simulink model "ros2webots_localization_model"  (R2023a)
settings: Solver=FixedStepAuto  StartTime=0.0  StopTime=inf  FixedStep=0.05  RelTol=1e-3  EnableMultiTasking=on
model workspace (MAT data in the model file):
  Logfile_Data_Object = robotics.ros.BagSelection
  Logfile_Data_Object.FilePath = '\\wsl.localhost\ubuntu\home\mjavadzallaghi\ros2_ws\ros2webots\baglog\rosbot_data_20240125_225927.bag'
  Logfile_Data_Object.StartTime = 1706210981.23
  Logfile_Data_Object.EndTime = 1706211126.25
  Logfile_Data_Object.NumMessages = 508
  Logfile_Data_Object.AvailableTopics = table
  Logfile_Data_Object.AvailableTopics.data{1} = [73; 435]
  Logfile_Data_Object.AvailableTopics.data{2} = categorical
  Logfile_Data_Object.AvailableTopics.data{2}.categoryNames = {'geometry_msgs/Twist'; 'sensor_msgs/Imu'}
  Logfile_Data_Object.AvailableTopics.data{2}.codes = [1; 2]
  Logfile_Data_Object.AvailableTopics.data{3}{1} = 'geometry_msgs/Vector3 Linear
    |   double X
    |   double Y
    |   double Z
    | geometry_msgs/Vector3 Angular
    |   double X
    |   double Y
    |   double Z
    | '
  Logfile_Data_Object.AvailableTopics.data{3}{2} = 'std_msgs/Header Header
    |   uint32 Seq
    |   Time Stamp
    |   char FrameId
    | geometry_msgs/Quaternion Orientation
    |   double X
    |   double Y
    |   double Z
    |   double W
    | double[9] OrientationCovariance
    | geometry_msgs/Vector3 AngularVelocity
    |   double X
    |   double Y
    |   double Z
    | double[9] AngularVelocityCovariance
    | geometry_msgs/Vector3 LinearAcceleration
    |   double X
    |   double Y
    |   double Z
    | double[9] LinearAccelerationCovariance
    | '
  Logfile_Data_Object.AvailableTopics.ndims = 2
  Logfile_Data_Object.AvailableTopics.nrows = 2
  Logfile_Data_Object.AvailableTopics.rownames = {'/webots/rosbot/command_vel'; '/webots/rosbot/imu'}
  Logfile_Data_Object.AvailableTopics.nvars = 3
  Logfile_Data_Object.AvailableTopics.varnames = {'NumMessages', 'MessageType', 'MessageDefinition'}
  Logfile_Data_Object.AvailableTopics.props.useVariableNamesOriginal = 0
  Logfile_Data_Object.AvailableTopics.props.useDimensionNamesOriginal = 0
  Logfile_Data_Object.AvailableTopics.props.CustomProps = struct()
  Logfile_Data_Object.AvailableTopics.props.VariableCustomProps = struct()
  Logfile_Data_Object.AvailableTopics.props.versionSavedFrom = 4
  Logfile_Data_Object.AvailableTopics.props.minCompatibleVersion = 1
  Logfile_Data_Object.AvailableTopics.props.incompatibilityMsg = ''
  Logfile_Data_Object.AvailableTopics.props.VersionSavedFrom = 4
  Logfile_Data_Object.AvailableTopics.props.Description = ''
  Logfile_Data_Object.AvailableTopics.props.VariableNamesOriginal = {}
  Logfile_Data_Object.AvailableTopics.props.DimensionNames = {'Row', 'Variables'}
  Logfile_Data_Object.AvailableTopics.props.DimensionNamesOriginal = {}
  Logfile_Data_Object.AvailableTopics.props.UserData = []
  Logfile_Data_Object.AvailableTopics.props.VariableDescriptions = {}
  Logfile_Data_Object.AvailableTopics.props.VariableUnits = {}
  Logfile_Data_Object.AvailableTopics.props.VariableContinuity = {}
  Logfile_Data_Object.MessageList = table
  Logfile_Data_Object.MessageList.data{1} = [1706210981.23 1706210981.23 1706210981.23 1706210983.05 1706210983.38 1706210983.7 1706210984.04 1706210984.38 1706210984.72 1706210985.07 1706210985.41 1706210985.73 ... (508 elements, 508x1)]
  Logfile_Data_Object.MessageList.data{2} = categorical
  Logfile_Data_Object.MessageList.data{2}.categoryNames = {'/webots/rosbot/command_vel'; '/webots/rosbot/imu'}
  Logfile_Data_Object.MessageList.data{2}.codes = [1; 1; 1; 2; 2; 2; 2; 2; 2; 2; 2; 1; 1; 1; 2; 2; 2; 2; 2; 2; 2; 2; 2; 2; 2; 2; 2; 2; 2; 2; 2; 2; 2; 2; 2; 2; 2; 2; 1; 1; 1; 2; 2; 2; 2; 2; 2; 2; 2; 2; 2; 2; 2; 2; 2; 2; 2; 2; 2; 2; 2; 2; 2; 2; 2; 2; 2; 1; 1; 1; 2; 2; 2; 2; 2; 2; 2; 2; 2; 2; 2; 2; 2; 2; 2; 2; 2; 2; 2; 2; 2; 1; 1; 1; 2; 2; 2; 2; 2; 2; 2; 2; 2; 2; 2; 2; 2; 2; 2; 2; 2; 2; 2; 2; 2; 2; 2; 2; 1; 1; 2; 1; 2; 2; 2; 2; 2; 2; 2; 2; 2; 2; 2; 2; 2; 2; 2; 2; 2; 2; 2; 2; 2; 2; 2; 2; 2; 2; 2; 2; 2; 2; 2; 2; 2; 2; 2; 2; 2; 2; 2; 2; 2; 2; 2; 2; 1; 1; 1; 2; 2; 2; 2; 2; 2; 2; 2; 2; 2; 2; 2; 2; 2; 2; 2; 2; 2; 2; 2; 2; 2; 2; 2; 1; 1; 1; 2; 2; 2; 2; 2; 2; 2; 2; 2; 2; 2; 2; 2; 2; 2; 2; 2; 2; 2; 2; 2; 2; 2; 2; 2; 2; 2; 1; 1; 1; 2; 2; 2; 2; 2; 2; 2; 2; 2; 2; 2; 2; 2; 2; 2; 2; 2; 2; 2; 2; 2; 2; 2; 2; 2; 2; 1; 1; 1; 2; 2; 2; 2; 2; 2; 2; 2; 2; 2; 2; 2; 2; 2; 2; 2; 2; 2; 2; 2; 1; 1; 1; 2; 2; 2; 2; 2; 2; 2; 2; 2; 2; 2; 2; 2; 2; 2; 2; 2; 2; 2; 2; 2; 2; 2; 2; 2; 1; 1; 1; 2; 2; 2; 2; 2; 2; 2; 1; 1; 2; 1; 2; 2; 2; 2; 2; 2; 1; 1; 1; 2; 2; 2; 2; 2; 2; 2; 2; 2; 2; 2; 2; 1; 1; 1; 2; 2; 2; 2; 2; 2; 2; 2; 2; 2; 2; 2; 2; 2; 2; 2; 2; 2; 2; 1; 1; 1; 2; 2; 2; 2; 2; 2; 2; 2; 2; 1; 1; 1; 2; 2; 2; 2; 2; 2; 2; 2; 2; 2; 2; 2; 1; 1; 1; 2; 2; 2; 2; 2; 2; 1; 1; 1; 2; 2; 2; 2; 2; 2; 2; 2; 2; 2; 2; 2; 1; 1; 1; 2; 2; 2; 2; 2; 2; 2; 2; 2; 2; 1; 1; 1; 2; 2; 2; 2; 2; 2; 2; 2; 2; 2; 1; 1; 1; 2; 2; 2; 2; 2; 2; 2; 1; 1; 1; 2; 2; 2; 2; 2; 2; 2; 2; 2; 2; 2; 2; 2; 2; 2; 2; 1; 1; 1; 2; 2; 2; 2; 2; 2; 2; 2; 2; 2; 2; 2; 2; 2; 2; 2; 1; 2; 2; 2; 2; 2; 2; 2; 2; 2; 2; 2; 2; 2; 2; 2; 2; 2; 2; 2; 2; 2; 2]
  Logfile_Data_Object.MessageList.data{3} = categorical
  Logfile_Data_Object.MessageList.data{3}.categoryNames = {'geometry_msgs/Twist'; 'sensor_msgs/Imu'}
  Logfile_Data_Object.MessageList.data{3}.codes = [1; 1; 1; 2; 2; 2; 2; 2; 2; 2; 2; 1; 1; 1; 2; 2; 2; 2; 2; 2; 2; 2; 2; 2; 2; 2; 2; 2; 2; 2; 2; 2; 2; 2; 2; 2; 2; 2; 1; 1; 1; 2; 2; 2; 2; 2; 2; 2; 2; 2; 2; 2; 2; 2; 2; 2; 2; 2; 2; 2; 2; 2; 2; 2; 2; 2; 2; 1; 1; 1; 2; 2; 2; 2; 2; 2; 2; 2; 2; 2; 2; 2; 2; 2; 2; 2; 2; 2; 2; 2; 2; 1; 1; 1; 2; 2; 2; 2; 2; 2; 2; 2; 2; 2; 2; 2; 2; 2; 2; 2; 2; 2; 2; 2; 2; 2; 2; 2; 1; 1; 2; 1; 2; 2; 2; 2; 2; 2; 2; 2; 2; 2; 2; 2; 2; 2; 2; 2; 2; 2; 2; 2; 2; 2; 2; 2; 2; 2; 2; 2; 2; 2; 2; 2; 2; 2; 2; 2; 2; 2; 2; 2; 2; 2; 2; 2; 1; 1; 1; 2; 2; 2; 2; 2; 2; 2; 2; 2; 2; 2; 2; 2; 2; 2; 2; 2; 2; 2; 2; 2; 2; 2; 2; 1; 1; 1; 2; 2; 2; 2; 2; 2; 2; 2; 2; 2; 2; 2; 2; 2; 2; 2; 2; 2; 2; 2; 2; 2; 2; 2; 2; 2; 2; 1; 1; 1; 2; 2; 2; 2; 2; 2; 2; 2; 2; 2; 2; 2; 2; 2; 2; 2; 2; 2; 2; 2; 2; 2; 2; 2; 2; 2; 1; 1; 1; 2; 2; 2; 2; 2; 2; 2; 2; 2; 2; 2; 2; 2; 2; 2; 2; 2; 2; 2; 2; 1; 1; 1; 2; 2; 2; 2; 2; 2; 2; 2; 2; 2; 2; 2; 2; 2; 2; 2; 2; 2; 2; 2; 2; 2; 2; 2; 2; 1; 1; 1; 2; 2; 2; 2; 2; 2; 2; 1; 1; 2; 1; 2; 2; 2; 2; 2; 2; 1; 1; 1; 2; 2; 2; 2; 2; 2; 2; 2; 2; 2; 2; 2; 1; 1; 1; 2; 2; 2; 2; 2; 2; 2; 2; 2; 2; 2; 2; 2; 2; 2; 2; 2; 2; 2; 1; 1; 1; 2; 2; 2; 2; 2; 2; 2; 2; 2; 1; 1; 1; 2; 2; 2; 2; 2; 2; 2; 2; 2; 2; 2; 2; 1; 1; 1; 2; 2; 2; 2; 2; 2; 1; 1; 1; 2; 2; 2; 2; 2; 2; 2; 2; 2; 2; 2; 2; 1; 1; 1; 2; 2; 2; 2; 2; 2; 2; 2; 2; 2; 1; 1; 1; 2; 2; 2; 2; 2; 2; 2; 2; 2; 2; 1; 1; 1; 2; 2; 2; 2; 2; 2; 2; 1; 1; 1; 2; 2; 2; 2; 2; 2; 2; 2; 2; 2; 2; 2; 2; 2; 2; 2; 1; 1; 1; 2; 2; 2; 2; 2; 2; 2; 2; 2; 2; 2; 2; 2; 2; 2; 2; 1; 2; 2; 2; 2; 2; 2; 2; 2; 2; 2; 2; 2; 2; 2; 2; 2; 2; 2; 2; 2; 2; 2]
  Logfile_Data_Object.MessageList.data{4} = [5438 5532 5626 5720 6078 6436 6794 7152 7510 7868 8226 8584 ... (508 elements, 508x1)]
  Logfile_Data_Object.MessageList.ndims = 2
  Logfile_Data_Object.MessageList.nrows = 508
  Logfile_Data_Object.MessageList.nvars = 4
  Logfile_Data_Object.MessageList.varnames = {'Time', 'Topic', 'MessageType', 'FileOffset'}
  Logfile_Data_Object.MessageList.props.useVariableNamesOriginal = 0
  Logfile_Data_Object.MessageList.props.useDimensionNamesOriginal = 0
  Logfile_Data_Object.MessageList.props.CustomProps = struct()
  Logfile_Data_Object.MessageList.props.VariableCustomProps = struct()
  Logfile_Data_Object.MessageList.props.versionSavedFrom = 4
  Logfile_Data_Object.MessageList.props.minCompatibleVersion = 1
  Logfile_Data_Object.MessageList.props.incompatibilityMsg = ''
  Logfile_Data_Object.MessageList.props.VersionSavedFrom = 4
  Logfile_Data_Object.MessageList.props.Description = ''
  Logfile_Data_Object.MessageList.props.VariableNamesOriginal = {}
  Logfile_Data_Object.MessageList.props.DimensionNames = {'Row', 'Variables'}
  Logfile_Data_Object.MessageList.props.DimensionNamesOriginal = {}
  Logfile_Data_Object.MessageList.props.UserData = []
  Logfile_Data_Object.MessageList.props.VariableDescriptions = {}
  Logfile_Data_Object.MessageList.props.VariableUnits = {}
  Logfile_Data_Object.MessageList.props.VariableContinuity = {}
  Logfile_Data_Object.RawMessageBuffer = containers.Map
  Logfile_Data_Object.RawMessageBuffer.serialization.keys = {}
  Logfile_Data_Object.RawMessageBuffer.serialization.values = {}
  Logfile_Data_Object.RawMessageBuffer.serialization.uniformity = 0
  Logfile_Data_Object.RawMessageBuffer.serialization.keyType = 'char'
  Logfile_Data_Object.RawMessageBuffer.serialization.valueType = 'any'
  Logfile_Data_Object.ImgMessageBuffer = containers.Map
  Logfile_Data_Object.ImgMessageBuffer.serialization.keys = {}
  Logfile_Data_Object.ImgMessageBuffer.serialization.values = {}
  Logfile_Data_Object.ImgMessageBuffer.serialization.uniformity = 0
  Logfile_Data_Object.ImgMessageBuffer.serialization.keyType = 'char'
  Logfile_Data_Object.ImgMessageBuffer.serialization.valueType = 'any'
  Logfile_Data_Object.PointCloudBuffer = containers.Map
  Logfile_Data_Object.PointCloudBuffer.serialization.keys = {}
  Logfile_Data_Object.PointCloudBuffer.serialization.values = {}
  Logfile_Data_Object.PointCloudBuffer.serialization.uniformity = 0
  Logfile_Data_Object.PointCloudBuffer.serialization.keyType = 'char'
  Logfile_Data_Object.PointCloudBuffer.serialization.valueType = 'any'
  Logfile_Data_Object.LaserScanBuffer = containers.Map
  Logfile_Data_Object.LaserScanBuffer.serialization.keys = {}
  Logfile_Data_Object.LaserScanBuffer.serialization.values = {}
  Logfile_Data_Object.LaserScanBuffer.serialization.uniformity = 0
  Logfile_Data_Object.LaserScanBuffer.serialization.keyType = 'char'
  Logfile_Data_Object.LaserScanBuffer.serialization.valueType = 'any'
  Logfile_Data_Object.TopicTypeMap = containers.Map
  Logfile_Data_Object.TopicTypeMap.serialization.keys = {'/webots/rosbot/command_vel', '/webots/rosbot/imu'}
  Logfile_Data_Object.TopicTypeMap.serialization.values = {'geometry_msgs/Twist', 'sensor_msgs/Imu'}
  Logfile_Data_Object.TopicTypeMap.serialization.uniformity = 1
  Logfile_Data_Object.TopicTypeMap.serialization.keyType = 'char'
  Logfile_Data_Object.TopicTypeMap.serialization.valueType = 'char'
  Logfile_Data_Object.TopicDefinitionMap = containers.Map
  Logfile_Data_Object.TopicDefinitionMap.serialization.keys = {'/webots/rosbot/command_vel', '/webots/rosbot/imu'}
  Logfile_Data_Object.TopicDefinitionMap.serialization.values{1} = 'geometry_msgs/Vector3 Linear
    |   double X
    |   double Y
    |   double Z
    | geometry_msgs/Vector3 Angular
    |   double X
    |   double Y
    |   double Z
    | '
  Logfile_Data_Object.TopicDefinitionMap.serialization.values{2} = 'std_msgs/Header Header
    |   uint32 Seq
    |   Time Stamp
    |   char FrameId
    | geometry_msgs/Quaternion Orientation
    |   double X
    |   double Y
    |   double Z
    |   double W
    | double[9] OrientationCovariance
    | geometry_msgs/Vector3 AngularVelocity
    |   double X
    |   double Y
    |   double Z
    | double[9] AngularVelocityCovariance
    | geometry_msgs/Vector3 LinearAcceleration
    |   double X
    |   double Y
    |   double Z
    | double[9] LinearAccelerationCovariance
    | '
  Logfile_Data_Object.TopicDefinitionMap.serialization.uniformity = 1
  Logfile_Data_Object.TopicDefinitionMap.serialization.keyType = 'char'
  Logfile_Data_Object.TopicDefinitionMap.serialization.valueType = 'char'
  Logfile_Data_Object.messageTypeMap = containers.Map
  Logfile_Data_Object.messageTypeMap.serialization.keys = {}
  Logfile_Data_Object.messageTypeMap.serialization.values = {}
  Logfile_Data_Object.messageTypeMap.serialization.uniformity = 0
  Logfile_Data_Object.messageTypeMap.serialization.keyType = 'char'
  Logfile_Data_Object.messageTypeMap.serialization.valueType = 'any'
  Logfile_Data_Object.Parser = robotics.ros.internal.tf.TransformationTreeParser
  Logfile_Data_Object.Parser.UseObjectMsg = 1
  Logfile_Path = '\\wsl.localhost\ubuntu\home\mjavadzallaghi\ros2_ws\ros2webots\baglog\rosbot_data_20240125_225927.bag'
  Logfile_Playback_Duration = nan
  Logfile_Playback_Offset = nan
libraries: robotlib x1
settings Model: Creator=MJava  LastModifiedBy=MJava
settings SolverCC: AllowMultiTaskInputOutput=on  AutoInsertRateTranBlk=on

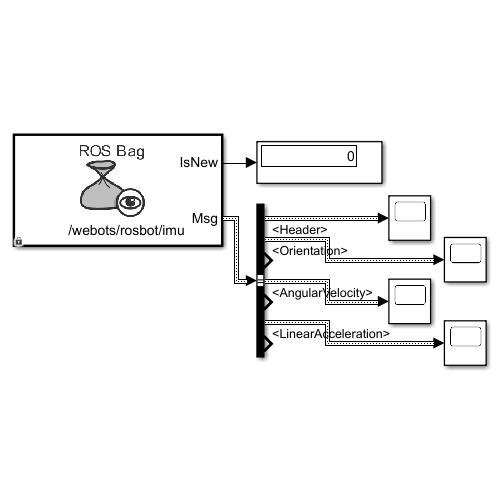
[thumbnail: Simulink's stored preview of the top-level diagram]
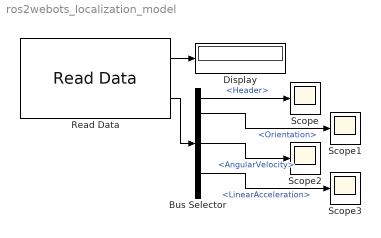
== system ros2webots_localization_model ==
  Bus Selector : BusSelector  OutputSignals=Header,Orientation,OrientationCovariance,AngularVelocity,AngularVelocityCovariance,LinearAcceleration,LinearAccelerationCovariance
  Display : Display
  Read Data : robotlib/Read Data  topic=/webots/rosbot/imu  sampleTime=-1  logfileType=rosbag  modelName=ros2webots_localization_model  msgType=sensor_msgs/Imu
  Scope{,1..3} (4 alike) : Scope
  wires:
  Read Data/2 -> Bus Selector/1
  Read Data/1 -> Display/1
  Bus Selector/1 -> Scope/1  "<Header>"
  Bus Selector/2 -> Scope1/1  "<Orientation>"
  Bus Selector/4 -> Scope2/1  "<AngularVelocity>"
  Bus Selector/6 -> Scope3/1  "<LinearAcceleration>"
